simulink model "zad2"  (R2016a)
settings: Solver=ode5  StartTime=0.0  StopTime=10.0  FixedStep=0.01  RelTol=1e-3
values from neighbouring files (symbols this model uses):
  b = 3    [zad1script.m]    (also in zad2script.m)
  k = acker(A,B,[-a -a])    [zad2script.m]
  L = acker(A',C2',[-3 -3])'    [zad2script.m]
  m = 1    [zad1script.m]    (also in zad2script.m)
  swD = 1    [zad1script.m]    (also in zad2script.m)
  swN = 1    [zad2script.m]
settings Model: Creator=milos  LastModifiedBy=milos

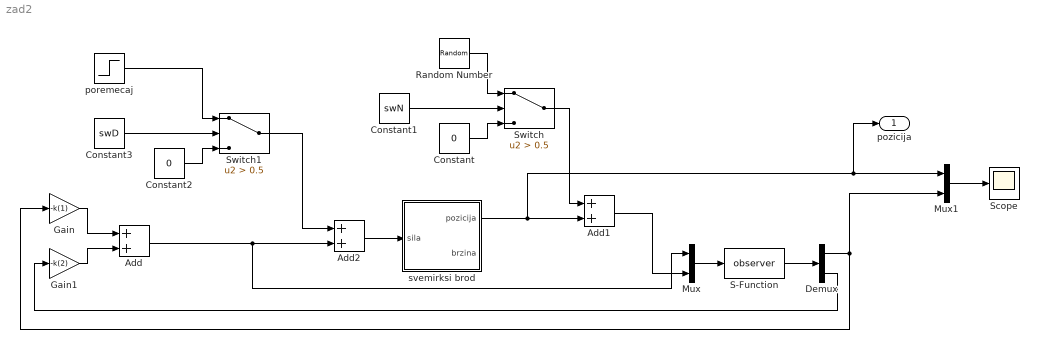
== system zad2 ==
  Add : Sum
  Add1 : Sum
  Add2 : Sum
  Constant : Constant  Value=0
  Constant1 : Constant  Value=swN
  Constant2 : Constant  Value=0
  Constant3 : Constant  Value=swD
  Demux : Demux  Outputs=2
  Gain : Gain  Gain=-k(1)
  Gain1 : Gain  Gain=-k(2)
  Mux : Mux  Inputs=2
  Mux1 : Mux  Inputs=2
  Random Number : RandomNumber  Variance=0.01
  S-Function : S-Function  FunctionName=observer  Parameters=b,m,L  SFunctionDeploymentMode=off  EnableBusSupport=off
  Scope : Scope
  Switch : Switch  Criteria=u2 > Threshold  Threshold=0.5
  Switch1 : Switch  Criteria=u2 > Threshold  Threshold=0.5
  poremecaj : Step  After=3  SampleTime=0
  svemirksi brod : Subsystem
  pozicija : Outport
  wires:
  Gain1/1 -> Add/2
  Gain/1 -> Add/1
  S-Function/1 -> Demux/1
  Demux/2 -> Gain1/1
  Demux/1 -> Gain/1, Mux1/2
  Mux/1 -> S-Function/1
  Mux1/1 -> Scope/1
  Random Number/1 -> Switch/1
  Constant/1 -> Switch/3
  Constant1/1 -> Switch/2
  Switch/1 -> Add1/1
  Add1/1 -> Mux/2
  svemirksi brod/1(pozicija) -> Add1/2, pozicija/1, Mux1/1
  Add2/1 -> svemirksi brod/1(sila)
  Add/1 -> Mux/1, Add2/2
  poremecaj/1 -> Switch1/1
  Constant2/1 -> Switch1/3
  Constant3/1 -> Switch1/2
  Switch1/1 -> Add2/1

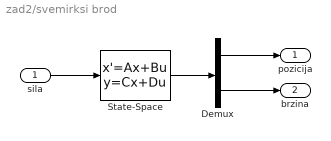
== system zad2/svemirksi brod ==
  sila : Inport
  Demux : Demux  Outputs=2
  State-Space : StateSpace  A=[0 1;0 -b/m]  B=[0;1/m]  C=[1 0; 0 1]  D=[0;0]  X0=[10;0]
  pozicija : Outport
  brzina : Outport  Port=2
  wires:
  State-Space/1 -> Demux/1
  sila/1 -> State-Space/1
  Demux/1 -> pozicija/1
  Demux/2 -> brzina/1
